simulink model "flightControlSystem"  (R2021a)
settings: Solver=ode3  StartTime=0  StopTime=TFinal  FixedStep=Ts  RelTol=1e-3  EnableMultiTasking=on
undefined symbols (not defined in the file): codertarget, Controller, DiscIntNeverNeededParam, Discrete, Estimator, g, gray, init, Sensors, Time, Ts, var_acc_angle_N, var_bias_gyr_N, var_gyro_p_N, Vehicle
libraries: simulink x39, pid_lib x4, ctrlSharedLib x4, sharedtransform x3, parrotlib x1
(part 3 of 4)

== matlab function flightControlSystem/Image Processing System/MATLAB Function ==
  data: in input; white_old input; all output; b output; x_new output; y_new output; x_old input; y_old input; change_old input; flag input; white output; flag2 input; change output; check_new output; check_old input; last input; last_old output
function [all,b,x_new,y_new,white,change,check_new,last_old] = calculate_ang(in,white_old, x_old, y_old, change_old, flag, flag2,check_old,last)
    white = 0;
    all = 0;
    red = in(:,:,1);
    filtered = imgaussfilt(red,2);
    b = imbinarize(filtered);
    for x=1:20
        for y=1:120
            b(y,x) = 0;
            b(y,(161-x)) = 0;
        end
    end
    N = 1;
    check_new = check_old;
    out = zeros(2,N);
    m00 = zeros(1,N);
    m01 = zeros(1,N);
    m10 = zeros(1,N);
    change = change_old; 
    % --------------------------------------------------------------

    if flag ~= 0
    
        m = -y_old/x_old;
        m1 = -1/m;
        %x = 1:160;
        %y = m1*x+c1;
     %----------------------------- Triangle 1
        
        x_tri1 = x_old*0.707 + y_old*-0.707;
        y_tri1 = x_old*0.707 + y_old*0.707;

        m = -y_tri1/x_tri1;
        m1 = -1/m;
        c1 = 60-80*m1;

        grad1 = m1;
        offset1 = c1;
        %[0.7071 0.7071; -0.7071 0.7071]
        x_tri2 = x_old*0.707 + y_old*0.707;
        y_tri2 = x_old*-0.707 + y_old*0.707;
        multiplier = 1;
        m = -y_tri2/x_tri2;
        m1 = -1/m;
        c1 = 60-80*m1;
        grad2 = m1;
        offset2 = c1;
        maxx = 70;
        limit = 2800;
        abs_grad = y_old/x_old;
            if abs_grad > 1 || abs_grad < -1
                if y_old > 0 
                    if x_old > 0 
                        last = 5;
                        if check_new == 0
                            change = 5;
                            if white_old ~=0
                                check_new = multiplier*maxx;
                            else
                                check_new = maxx;
                            end
                        end
                        if change ~= last
                            %change = last;
                            check_new = check_new - 1;
                        elseif change == last
                            if check_new < maxx
                                check_new = check_new + 1;
                            end
                        end
                        
                        if change == 0 %FRFC Row then Col
                            for row=1:120
                                for col=1:160
                                    if row>grad1*col + offset1 || row>grad2*col + offset2
                                        if b(row,col) == 1 && white < limit && flag2 == 1
                                            b(row,col) = 0;
                                            white = white + 1;
                                            all = all + 1;
                                        elseif b(row,col) == 1
                                            all = all + 1;
                                        end
                                    end
                                end
                            end
                        elseif change == 1  %FRFC Col then Row
                            for col=1:160
                                for row=1:120
                                    if row>grad1*col + offset1 || row>grad2*col + offset2
                                        if b(row,col) == 1 && white < limit && flag2 == 1
                                            b(row,col) = 0;
                                            white = white + 1;
                                            all = all + 1;
                                        elseif b(row,col) == 1
                                            all = all + 1;
                                        end
                                    end
                                end
                            end
                        elseif change == 2  %FRLC Row then Col
                            for row=1:120
                                for col=1:160
                                    if row>grad1*(161-col) + offset1 || row>grad2*(161-col) + offset2
                                         if b(row,(161-col)) == 1 && white < limit && flag2 == 1
                                            b(row,(161-col)) = 0;
                                            white = white + 1;
                                            all = all + 1;
                                         elseif b(row,(161-col)) == 1
                                            all = all + 1;
                                        end
                                    end
                                end
                            end
                            
                            
                         elseif change == 3  %FRLC Col then Row
                            for col=1:160
                                for row=1:120
                                    if row>grad1*(161-col) + offset1 || row>grad2*(161-col) + offset2
                                         if b(row,(161-col)) == 1 && white < limit && flag2 == 1
                                            b(row,(161-col)) = 0;
                                            white = white + 1;
                                            all = all + 1;
                                         elseif b(row,(161-col)) == 1
                                            all = all + 1;
                                        end
                                    end
                                end
                            end  
                           
                            
                          elseif change == 4  %LRFC Row then Col
                            for row=1:120
                                for col=1:160
                                    if (121-row)>grad1*col + offset1 || (121-row)>grad2*col + offset2
                                         if b((121-row),col) == 1 && white < limit && flag2 == 1
                                            b((121-row),col) = 0;
                                            white = white + 1;
                                            all = all + 1;
                                         elseif b((121-row),col) == 1
                                            all = all + 1;
                                        end
                                    end
                                end
                            end  
                            
                          elseif change == 5  %LRFC Col then Row
                            for col=1:160
                                for row=1:120
                                    if (121-row)>grad1*col + offset1 || (121-row)>grad2*col + offset2
                                         if b((121-row),col) == 1 && white < limit && flag2 == 1
                                            b((121-row),col) = 0;
                                            white = white + 1;
                                            all = all + 1;
                                         elseif b((121-row),col) == 1
                                            all = all + 1;
                                        end
                                    end
                                end
                            end  
                            
                           elseif change == 6  %LRLC Row then Col
                            for row=1:120
                                for col=1:160
                                    if (121-row)>grad1*(161-col) + offset1 || (121-row)>grad2*(161-col) + offset2
                                         if b((121-row),(161-col)) == 1 && white < limit && flag2 == 1
                                            b((121-row),(161-col)) = 0;
                                            white = white + 1;
                                            all = all + 1;
                                         elseif b((121-row),(161-col)) == 1
                                            all = all + 1;
                                        end
                                    end
                                end
                            end  
                            
                            elseif change == 7  %LRLC Col then Row
                            for col=1:160
                                for row=1:120
                                    if (121-row)>grad1*(161-col) + offset1 || (121-row)>grad2*(161-col) + offset2
                                         if b((121-row),(161-col)) == 1 && white < limit && flag2 == 1
                                            b((121-row),(161-col)) = 0;
                                            white = white + 1;
                                            all = all + 1;
                                         elseif b((121-row),(161-col)) == 1
                                            all = all + 1;
                                        end
                                    end
                                end
                            end   
                        end
                    else
                        last = 7;
                        if check_new == 0
                            if white_old ~=0
                                check_new = multiplier*maxx;
                            else
                                check_new = maxx;
                            end
                            change = 7;
                        end
                        if change ~= last
                            check_new = check_new - 1;
                            %change = last;
                        elseif change == last
                            if check_new < maxx
                                check_new = check_new + 1;
                            end
                        end
                        

                        
                        if change == 0 %FRFC Row then Col
                            for row=1:120
                                for col=1:160
                                    if row>grad1*col + offset1 || row>grad2*col + offset2
                                        if b(row,col) == 1 && white < limit && flag2 == 1
                                            b(row,col) = 0;
                                            white = white + 1;
                                            all = all + 1;
                                        elseif b(row,col) == 1
                                            all = all + 1;
                                        end
                                    end
                                end
                            end
                        elseif change == 1  %FRFC Col then Row
                            for col=1:160
                                for row=1:120
                                    if row>grad1*col + offset1 || row>grad2*col + offset2
                                        if b(row,col) == 1 && white < limit && flag2 == 1
                                            b(row,col) = 0;
                                            white = white + 1;
                                            all = all + 1;
                                        elseif b(row,col) == 1
                                            all = all + 1;
                                        end
                                    end
                                end
                            end
                        elseif change == 2  %FRLC Row then Col
                            for row=1:120
                                for col=1:160
                                    if row>grad1*(161-col) + offset1 || row>grad2*(161-col) + offset2
                                         if b(row,(161-col)) == 1 && white < limit && flag2 == 1
                                            b(row,(161-col)) = 0;
                                            white = white + 1;
                                            all = all + 1;
                                         elseif b(row,(161-col)) == 1
                                            all = all + 1;
                                        end
                                    end
                                end
                            end
                            
                            
                         elseif change == 3  %FRLC Col then Row
                            for col=1:160
                                for row=1:120
                                    if row>grad1*(161-col) + offset1 || row>grad2*(161-col) + offset2
                                         if b(row,(161-col)) == 1 && white < limit && flag2 == 1
                                            b(row,(161-col)) = 0;
                                            white = white + 1;
                                            all = all + 1;
                                         elseif b(row,(161-col)) == 1
                                            all = all + 1;
                                        end
                                    end
                                end
                            end  
                           
                            
                          elseif change == 4  %LRFC Row then Col
                            for row=1:120
                                for col=1:160
                                    if (121-row)>grad1*col + offset1 || (121-row)>grad2*col + offset2
                                         if b((121-row),col) == 1 && white < limit && flag2 == 1
                                            b((121-row),col) = 0;
                                            white = white + 1;
                                            all = all + 1;
                                         elseif b((121-row),col) == 1
                                            all = all + 1;
                                        end
                                    end
                                end
                            end  
                            
                          elseif change == 5  %LRFC Col then Row
                            for col=1:160
                                for row=1:120
                                    if (121-row)>grad1*col + offset1 || (121-row)>grad2*col + offset2
                                         if b((121-row),col) == 1 && white < limit && flag2 == 1
                                            b((121-row),col) = 0;
                                            white = white + 1;
                                            all = all + 1;
                                         elseif b((121-row),col) == 1
                                            all = all + 1;
                                        end
                                    end
                                end
                            end  
                            
                           elseif change == 6  %LRLC Row then Col
                            for row=1:120
                                for col=1:160
                                    if (121-row)>grad1*(161-col) + offset1 || (121-row)>grad2*(161-col) + offset2
                                         if b((121-row),(161-col)) == 1 && white < limit && flag2 == 1
                                            b((121-row),(161-col)) = 0;
                                            white = white + 1;
                                            all = all + 1;
                                         elseif b((121-row),(161-col)) == 1
                                            all = all + 1;
                                        end
                                    end
                                end
                            end  
                            
                            elseif change == 7  %LRLC Col then Row
                            for col=1:160
                                for row=1:120
                                    if (121-row)>grad1*(161-col) + offset1 || (121-row)>grad2*(161-col) + offset2
                                         if b((121-row),(161-col)) == 1 && white < limit && flag2 == 1
                                            b((121-row),(161-col)) = 0;
                                            white = white + 1;
                                            all = all + 1;
                                         elseif b((121-row),(161-col)) == 1
                                            all = all + 1;
                                        end
                                    end
                                end
                            end
                        end 
                    end
                else
                    if x_old > 0
                        
                        last = 1;
                        if check_new == 0
                            change = 1;
                            if white_old ~=0
                                check_new = multiplier*maxx;
                            else
                                check_new = maxx;
                            end
                        end
                        if change ~= last
                            check_new = check_new - 1;
                            %change = last;
                        elseif change == last
                            if check_new < maxx
                                check_new = check_new + 1;
                            end
                        end
                        
                        

                        if change == 0 %FRFC Row then Col
                            for row=1:120
                                for col=1:160
                                    if row<grad1*col + offset1 || row<grad2*col + offset2
                                        if b(row,col) == 1 && white < limit && flag2 == 1
                                            b(row,col) = 0;
                                            white = white + 1;
                                            all = all + 1;
                                        elseif b(row,col) == 1
                                            all = all + 1;
                                        end
                                    end
                                end
                            end
                        elseif change == 1  %FRFC Col then Row
                            for col=1:160
                                for row=1:120
                                    if row<grad1*col + offset1 || row<grad2*col + offset2
                                        if b(row,col) == 1 && white < limit && flag2 == 1
                                            b(row,col) = 0;
                                            white = white + 1;
                                            all = all + 1;
                                        elseif b(row,col) == 1
                                            all = all + 1;
                                        end
                                    end
                                end
                            end
                        elseif change == 2  %FRLC Row then Col
                            for row=1:120
                                for col=1:160
                                    if row<grad1*(161-col) + offset1 || row<grad2*(161-col) + offset2
                                         if b(row,(161-col)) == 1 && white < limit && flag2 == 1
                                            b(row,(161-col)) = 0;
                                            white = white + 1;
                                            all = all + 1;
                                         elseif b(row,(161-col)) == 1
                                            all = all + 1;
                                        end
                                    end
                                end
                            end
                            
                            
                         elseif change == 3  %FRLC Col then Row
                            for col=1:160
                                for row=1:120
                                    if row<grad1*(161-col) + offset1 || row<grad2*(161-col) + offset2
                                         if b(row,(161-col)) == 1 && white < limit && flag2 == 1
                                            b(row,(161-col)) = 0;
                                            white = white + 1;
                                            all = all + 1;
                                         elseif b(row,(161-col)) == 1
                                            all = all + 1;
                                        end
                                    end
                                end
                            end  
                           
                            
                          elseif change == 4  %LRFC Row then Col
                            for row=1:120
                                for col=1:160
                                    if (121-row)<grad1*col + offset1 || (121-row)<grad2*col + offset2
                                         if b((121-row),col) == 1 && white < limit && flag2 == 1
                                            b((121-row),col) = 0;
                                            white = white + 1;
                                            all = all + 1;
                                         elseif b((121-row),col) == 1
                                            all = all + 1;
                                        end
                                    end
                                end
                            end  
                            
                          elseif change == 5  %LRFC Col then Row
                            for col=1:160
                                for row=1:120
                                    if (121-row)<grad1*col + offset1 || (121-row)<grad2*col + offset2
                                         if b((121-row),col) == 1 && white < limit && flag2 == 1
                                            b((121-row),col) = 0;
                                            white = white + 1;
                                            all = all + 1;
                                         elseif b((121-row),col) == 1
                                            all = all + 1;
                                        end
                                    end
                                end
                            end  
                            
                           elseif change == 6  %LRLC Row then Col
                            for row=1:120
                                for col=1:160
                                    if (121-row)<grad1*(161-col) + offset1 || (121-row)<grad2*(161-col) + offset2
                                         if b((121-row),(161-col)) == 1 && white < limit && flag2 == 1
                                            b((121-row),(161-col)) = 0;
                                            white = white + 1;
                                            all = all + 1;
                                         elseif b((121-row),(161-col)) == 1
                                            all = all + 1;
                                        end
                                    end
                                end
                            end  
                            
                            elseif change == 7  %LRLC Col then Row
                            for col=1:160
                                for row=1:120
                                    if (121-row)<grad1*(161-col) + offset1 || (121-row)<grad2*(161-col) + offset2
                                         if b((121-row),(161-col)) == 1 && white < limit && flag2 == 1
                                            b((121-row),(161-col)) = 0;
                                            white = white + 1;
                                            all = all + 1;
                                         elseif b((121-row),(161-col)) == 1
                                            all = all + 1;
                                        end
                                    end
                                end
                            end
                        end  
                        
                        
 
                        
                        
                    else
                        
                        last = 3;
                        if check_new == 0
                            change = 3;
                            if white_old ~=0
                                check_new = multiplier*maxx;
                            else
                                check_new = maxx;
                            end
                        end
                        if change ~= last
                            check_new = check_new - 1;
                            %change = last;
                        elseif change == last
                            if check_new < maxx
                                check_new = check_new + 1;
                            end
                        end
                        
                        
                        
                        
                        if change == 0 %FRFC Row then Col
                            for row=1:120
                                for col=1:160
                                    if row<grad1*col + offset1 || row<grad2*col + offset2
                                        if b(row,col) == 1 && white < limit && flag2 == 1
                                            b(row,col) = 0;
                                            white = white + 1;
                                            all = all + 1;
                                        elseif b(row,col) == 1
                                            all = all + 1;
                                        end
                                    end
                                end
                            end
                        elseif change == 1  %FRFC Col then Row
                            for col=1:160
                                for row=1:120
                                    if row<grad1*col + offset1 || row<grad2*col + offset2
                                        if b(row,col) == 1 && white < limit && flag2 == 1
                                            b(row,col) = 0;
                                            white = white + 1;
                                            all = all + 1;
                                        elseif b(row,col) == 1
                                            all = all + 1;
                                        end
                                    end
                                end
                            end
                        elseif change == 2  %FRLC Row then Col
                            for row=1:120
                                for col=1:160
                                    if row<grad1*(161-col) + offset1 || row<grad2*(161-col) + offset2
                                         if b(row,(161-col)) == 1 && white < limit && flag2 == 1
                                            b(row,(161-col)) = 0;
                                            white = white + 1;
                                            all = all + 1;
                                         elseif b(row,(161-col)) == 1
                                            all = all + 1;
                                        end
                                    end
                                end
                            end
                            
                            
                         elseif change == 3  %FRLC Col then Row
                            for col=1:160
                                for row=1:120
                                    if row<grad1*(161-col) + offset1 || row<grad2*(161-col) + offset2
                                         if b(row,(161-col)) == 1 && white < limit && flag2 == 1
                                            b(row,(161-col)) = 0;
                                            white = white + 1;
                                            all = all + 1;
                                         elseif b(row,(161-col)) == 1
                                            all = all + 1;
                                        end
                                    end
                                end
                            end  
                           
                            
                          elseif change == 4  %LRFC Row then Col
                            for row=1:120
                                for col=1:160
                                    if (121-row)<grad1*col + offset1 || (121-row)<grad2*col + offset2
                                         if b((121-row),col) == 1 && white < limit && flag2 == 1
                                            b((121-row),col) = 0;
                                            white = white + 1;
                                            all = all + 1;
                                         elseif b((121-row),col) == 1
                                            all = all + 1;
                                        end
                                    end
                                end
                            end  
                            
                          elseif change == 5  %LRFC Col then Row
                            for col=1:160
                                for row=1:120
                                    if (121-row)<grad1*col + offset1 || (121-row)<grad2*col + offset2
                                         if b((121-row),col) == 1 && white < limit && flag2 == 1
                                            b((121-row),col) = 0;
                                            white = white + 1;
                                            all = all + 1;
                                         elseif b((121-row),col) == 1
                                            all = all + 1;
                                        end
                                    end
                                end
                            end  
                            
                           elseif change == 6  %LRLC Row then Col
                            for row=1:120
                                for col=1:160
                                    if (121-row)<grad1*(161-col) + offset1 || (121-row)<grad2*(161-col) + offset2
                                         if b((121-row),(161-col)) == 1 && white < limit && flag2 == 1
                                            b((121-row),(161-col)) = 0;
                                            white = white + 1;
                                            all = all + 1;
                                         elseif b((121-row),(161-col)) == 1
                                            all = all + 1;
                                        end
                                    end
                                end
                            end  
                            
                            elseif change == 7  %LRLC Col then Row
                            for col=1:160
                                for row=1:120
                                    if (121-row)<grad1*(161-col) + offset1 || (121-row)<grad2*(161-col) + offset2
                                         if b((121-row),(161-col)) == 1 && white < limit && flag2 == 1
                                            b((121-row),(161-col)) = 0;
                                            white = white + 1;
                                            all = all + 1;
                                         elseif b((121-row),(161-col)) == 1
                                            all = all + 1;
                                        end
                                    end
                                end
                            end
                        end 
                                     
                        
                    end
                end
            else
                if x_old > 0
                    if y_old < 0
                        last = 0;
                        if check_new == 0
                            change = 0;
                            if white_old ~=0
                                check_new = multiplier*maxx;
                            else
                                check_new = maxx;
                            end
                        end
                        if change ~= last
                            %change = last;
                            check_new = check_new - 1;
                        elseif change == last
                            if check_new < maxx
                                check_new = check_new + 1;
                            end
                        end
                        
                        
                        
                        
                        if change == 0 %FRFC Row then Col
                            for row=1:120
                                for col=1:160
                                    if row>grad1*col + offset1 || row<grad2*col + offset2
                                        if b(row,col) == 1 && white < limit && flag2 == 1
                                            b(row,col) = 0;
                                            white = white + 1;
                                            all = all + 1;
                                        elseif b(row,col) == 1
                                            all = all + 1;
                                        end
                                    end
                                end
                            end
                        elseif change == 1  %FRFC Col then Row
                            for col=1:160
                                for row=1:120
                                    if row>grad1*col + offset1 || row<grad2*col + offset2
                                        if b(row,col) == 1 && white < limit && flag2 == 1
                                            b(row,col) = 0;
                                            white = white + 1;
                                            all = all + 1;
                                        elseif b(row,col) == 1
                                            all = all + 1;
                                        end
                                    end
                                end
                            end
                        elseif change == 2  %FRLC Row then Col
                            for row=1:120
                                for col=1:160
                                    if row>grad1*(161-col) + offset1 || row<grad2*(161-col) + offset2
                                         if b(row,(161-col)) == 1 && white < limit && flag2 == 1
                                            b(row,(161-col)) = 0;
                                            white = white + 1;
                                            all = all + 1;
                                         elseif b(row,(161-col)) == 1
                                            all = all + 1;
                                        end
                                    end
                                end
                            end
                            
                            
                         elseif change == 3  %FRLC Col then Row
                            for col=1:160
                                for row=1:120
                                    if row>grad1*(161-col) + offset1 || row<grad2*(161-col) + offset2
                                         if b(row,(161-col)) == 1 && white < limit && flag2 == 1
                                            b(row,(161-col)) = 0;
                                            white = white + 1;
                                            all = all + 1;
                                         elseif b(row,(161-col)) == 1
                                            all = all + 1;
                                        end
                                    end
                                end
                            end  
                           
                            
                          elseif change == 4  %LRFC Row then Col
                            for row=1:120
                                for col=1:160
                                    if (121-row)>grad1*col + offset1 || (121-row)<grad2*col + offset2
                                         if b((121-row),col) == 1 && white < limit && flag2 == 1
                                            b((121-row),col) = 0;
                                            white = white + 1;
                                            all = all + 1;
                                         elseif b((121-row),col) == 1
                                            all = all + 1;
                                        end
                                    end
                                end
                            end  
                            
                          elseif change == 5  %LRFC Col then Row
                            for col=1:160
                                for row=1:120
                                    if (121-row)>grad1*col + offset1 || (121-row)<grad2*col + offset2
                                         if b((121-row),col) == 1 && white < limit && flag2 == 1
                                            b((121-row),col) = 0;
                                            white = white + 1;
                                            all = all + 1;
                                         elseif b((121-row),col) == 1
                                            all = all + 1;
                                        end
                                    end
                                end
                            end  
                            
                           elseif change == 6  %LRLC Row then Col
                            for row=1:120
                                for col=1:160
                                    if (121-row)>grad1*(161-col) + offset1 || (121-row)<grad2*(161-col) + offset2
                                         if b((121-row),(161-col)) == 1 && white < limit && flag2 == 1
                                            b((121-row),(161-col)) = 0;
                                            white = white + 1;
                                            all = all + 1;
                                         elseif b((121-row),(161-col)) == 1
                                            all = all + 1;
                                        end
                                    end
                                end
                            end  
                            
                            elseif change == 7  %LRLC Col then Row
                            for col=1:160
                                for row=1:120
                                    if (121-row)>grad1*(161-col) + offset1 || (121-row)<grad2*(161-col) + offset2
                                         if b((121-row),(161-col)) == 1 && white < limit && flag2 == 1
                                            b((121-row),(161-col)) = 0;
                                            white = white + 1;
                                            all = all + 1;
                                         elseif b((121-row),(161-col)) == 1
                                            all = all + 1;
                                        end
                                    end
                                end
                            end
                        end 
                        
                        
                        
                        
                        
                    else
                        
                        last = 4;
                        if check_new == 0
                            change = 4;
                            if white_old ~=0
                                check_new = multiplier*maxx;
                            else
                                check_new = maxx;
                            end
                        end
                        if change ~= last
                            %change = last;
                            check_new = check_new - 1;
                        elseif change == last
                            if check_new < maxx
                                check_new = check_new + 1;
                            end
                        end
                        
                        if change == 0 %FRFC Row then Col
                            for row=1:120
                                for col=1:160
                                    if row>grad1*col + offset1 || row<grad2*col + offset2
                                        if b(row,col) == 1 && white < limit && flag2 == 1
                                            b(row,col) = 0;
                                            white = white + 1;
                                            all = all + 1;
                                        elseif b(row,col) == 1
                                            all = all + 1;
                                        end
                                    end
                                end
                            end
                        elseif change == 1  %FRFC Col then Row
                            for col=1:160
                                for row=1:120
                                    if row>grad1*col + offset1 || row<grad2*col + offset2
                                        if b(row,col) == 1 && white < limit && flag2 == 1
                                            b(row,col) = 0;
                                            white = white + 1;
                                            all = all + 1;
                                        elseif b(row,col) == 1
                                            all = all + 1;
                                        end
                                    end
                                end
                            end
                        elseif change == 2  %FRLC Row then Col
                            for row=1:120
                                for col=1:160
                                    if row>grad1*(161-col) + offset1 || row<grad2*(161-col) + offset2
                                         if b(row,(161-col)) == 1 && white < limit && flag2 == 1
                                            b(row,(161-col)) = 0;
                                            white = white + 1;
                                            all = all + 1;
                                         elseif b(row,(161-col)) == 1
                                            all = all + 1;
                                        end
                                    end
                                end
                            end
                            
                            
                         elseif change == 3  %FRLC Col then Row
                            for col=1:160
                                for row=1:120
                                    if row>grad1*(161-col) + offset1 || row<grad2*(161-col) + offset2
                                         if b(row,(161-col)) == 1 && white < limit && flag2 == 1
                                            b(row,(161-col)) = 0;
                                            white = white + 1;
                                            all = all + 1;
                                         elseif b(row,(161-col)) == 1
                                            all = all + 1;
                                        end
                                    end
                                end
                            end  
                           
                            
                          elseif change == 4  %LRFC Row then Col
                            for row=1:120
                                for col=1:160
                                    if (121-row)>grad1*col + offset1 || (121-row)<grad2*col + offset2
                                         if b((121-row),col) == 1 && white < limit && flag2 == 1
                                            b((121-row),col) = 0;
                                            white = white + 1;
                                            all = all + 1;
                                         elseif b((121-row),col) == 1
                                            all = all + 1;
                                        end
                                    end
                                end
                            end  
                            
                          elseif change == 5  %LRFC Col then Row
                            for col=1:160
                                for row=1:120
                                    if (121-row)>grad1*col + offset1 || (121-row)<grad2*col + offset2
                                         if b((121-row),col) == 1 && white < limit && flag2 == 1
                                            b((121-row),col) = 0;
                                            white = white + 1;
                                            all = all + 1;
                                         elseif b((121-row),col) == 1
                                            all = all + 1;
                                        end
                                    end
                                end
                            end  
                            
                           elseif change == 6  %LRLC Row then Col
                            for row=1:120
                                for col=1:160
                                    if (121-row)>grad1*(161-col) + offset1 || (121-row)<grad2*(161-col) + offset2
                                         if b((121-row),(161-col)) == 1 && white < limit && flag2 == 1
                                            b((121-row),(161-col)) = 0;
                                            white = white + 1;
                                            all = all + 1;
                                         elseif b((121-row),(161-col)) == 1
                                            all = all + 1;
                                        end
                                    end
                                end
                            end  
                            
                            elseif change == 7  %LRLC Col then Row
                            for col=1:160
                                for row=1:120
                                    if (121-row)>grad1*(161-col) + offset1 || (121-row)<grad2*(161-col) + offset2
                                         if b((121-row),(161-col)) == 1 && white < limit && flag2 == 1
                                            b((121-row),(161-col)) = 0;
                                            white = white + 1;
                                            all = all + 1;
                                         elseif b((121-row),(161-col)) == 1
                                            all = all + 1;
                                        end
                                    end
                                end
                            end
                        end           
                   
                    end
                else
                    if y_old < 0
                        
                        last = 2;
                        if check_new == 0
                            change = 2;
                            if white_old ~=0
                                check_new = multiplier*maxx;
                            else
                                check_new = maxx;
                            end
                        end
                        if change ~= last
                            %change = last;
                            check_new = check_new - 1;
                        elseif change == last
                            if check_new < maxx
                                check_new = check_new + 1;
                            end
                        end
                        
                        if change == 0 %FRFC Row then Col
                            for row=1:120
                                for col=1:160
                                    if row<grad1*col + offset1 || row>grad2*col + offset2
                                        if b(row,col) == 1 && white < limit && flag2 == 1
                                            b(row,col) = 0;
                                            white = white + 1;
                                            all = all + 1;
                                        elseif b(row,col) == 1
                                            all = all + 1;
                                        end
                                    end
                                end
                            end
                        elseif change == 1  %FRFC Col then Row
                            for col=1:160
                                for row=1:120
                                    if row<grad1*col + offset1 || row>grad2*col + offset2
                                        if b(row,col) == 1 && white < limit && flag2 == 1
                                            b(row,col) = 0;
                                            white = white + 1;
                                            all = all + 1;
                                        elseif b(row,col) == 1
                                            all = all + 1;
                                        end
                                    end
                                end
                            end
                        elseif change == 2  %FRLC Row then Col
                            for row=1:120
                                for col=1:160
                                    if row<grad1*(161-col) + offset1 || row>grad2*(161-col) + offset2
                                         if b(row,(161-col)) == 1 && white < limit && flag2 == 1
                                            b(row,(161-col)) = 0;
                                            white = white + 1;
                                            all = all + 1;
                                         elseif b(row,(161-col)) == 1
                                            all = all + 1;
                                        end
                                    end
                                end
                            end
                            
                            
                         elseif change == 3  %FRLC Col then Row
                            for col=1:160
                                for row=1:120
                                    if row<grad1*(161-col) + offset1 || row>grad2*(161-col) + offset2
                                         if b(row,(161-col)) == 1 && white < limit && flag2 == 1
                                            b(row,(161-col)) = 0;
                                            white = white + 1;
                                            all = all + 1;
                                         elseif b(row,(161-col)) == 1
                                            all = all + 1;
                                        end
                                    end
                                end
                            end  
                           
                            
                          elseif change == 4  %LRFC Row then Col
                            for row=1:120
                                for col=1:160
                                    if (121-row)<grad1*col + offset1 || (121-row)>grad2*col + offset2
                                         if b((121-row),col) == 1 && white < limit && flag2 == 1
                                            b((121-row),col) = 0;
                                            white = white + 1;
                                            all = all + 1;
                                         elseif b((121-row),col) == 1
                                            all = all + 1;
                                        end
                                    end
                                end
                            end  
                            
                          elseif change == 5  %LRFC Col then Row
                            for col=1:160
                                for row=1:120
                                    if (121-row)<grad1*col + offset1 || (121-row)>grad2*col + offset2
                                         if b((121-row),col) == 1 && white < limit && flag2 == 1
                                            b((121-row),col) = 0;
                                            white = white + 1;
                                            all = all + 1;
                                         elseif b((121-row),col) == 1
                                            all = all + 1;
                                        end
                                    end
                                end
                            end  
                            
                           elseif change == 6  %LRLC Row then Col
                            for row=1:120
                                for col=1:160
                                    if (121-row)<grad1*(161-col) + offset1 || (121-row)>grad2*(161-col) + offset2
                                         if b((121-row),(161-col)) == 1 && white < limit && flag2 == 1
                                            b((121-row),(161-col)) = 0;
                                            white = white + 1;
                                            all = all + 1;
                                         elseif b((121-row),(161-col)) == 1
                                            all = all + 1;
                                        end
                                    end
                                end
                            end  
                            
                            elseif change == 7  %LRLC Col then Row
                            for col=1:160
                                for row=1:120
                                    if (121-row)<grad1*(161-col) + offset1 || (121-row)>grad2*(161-col) + offset2
                                         if b((121-row),(161-col)) == 1 && white < limit && flag2 == 1
                                            b((121-row),(161-col)) = 0;
                                            white = white + 1;
                                            all = all + 1;
                                         elseif b((121-row),(161-col)) == 1
                                            all = all + 1;
                                        end
                                    end
                                end
                            end
                        end 
                       
                        
                    else
                        last = 6;
                        if check_new == 0
                            change = 6;
                            if white_old ~=0
                                check_new = multiplier*maxx;
                            else
                                check_new = maxx;
                            end
                        end
                        if change ~= last
                            check_new = check_new - 1;
                            %change = last;
                        elseif change == last
                            if check_new < maxx
                                check_new = check_new + 1;
                            end
                        end
                        
                        if change == 0 %FRFC Row then Col
                            for row=1:120
                                for col=1:160
                                    if row<grad1*col + offset1 || row>grad2*col + offset2
                                        if b(row,col) == 1 && white < limit && flag2 == 1
                                            b(row,col) = 0;
                                            white = white + 1;
                                            all = all + 1;
                                        elseif b(row,col) == 1
                                            all = all + 1;
                                        end
                                    end
                                end
                            end
                        elseif change == 1  %FRFC Col then Row
                            for col=1:160
                                for row=1:120
                                    if row<grad1*col + offset1 || row>grad2*col + offset2
                                        if b(row,col) == 1 && white < limit && flag2 == 1
                                            b(row,col) = 0;
                                            white = white + 1;
                                            all = all + 1;
                                        elseif b(row,col) == 1
                                            all = all + 1;
                                        end
                                    end
                                end
                            end
                        elseif change == 2  %FRLC Row then Col
                            for row=1:120
                                for col=1:160
                                    if row<grad1*(161-col) + offset1 || row>grad2*(161-col) + offset2
                                         if b(row,(161-col)) == 1 && white < limit && flag2 == 1
                                            b(row,(161-col)) = 0;
                                            white = white + 1;
                                            all = all + 1;
                                         elseif b(row,(161-col)) == 1
                                            all = all + 1;
                                        end
                                    end
                                end
                            end
                            
                            
                         elseif change == 3  %FRLC Col then Row
                            for col=1:160
                                for row=1:120
                                    if row<grad1*(161-col) + offset1 || row>grad2*(161-col) + offset2
                                         if b(row,(161-col)) == 1 && white < limit && flag2 == 1
                                            b(row,(161-col)) = 0;
                                            white = white + 1;
                                            all = all + 1;
                                         elseif b(row,(161-col)) == 1
                                            all = all + 1;
                                        end
                                    end
                                end
                            end  
                           
                            
                          elseif change == 4  %LRFC Row then Col
                            for row=1:120
                                for col=1:160
                                    if (121-row)<grad1*col + offset1 || (121-row)>grad2*col + offset2
                                         if b((121-row),col) == 1 && white < limit && flag2 == 1
                                            b((121-row),col) = 0;
                                            white = white + 1;
                                            all = all + 1;
                                         elseif b((121-row),col) == 1
                                            all = all + 1;
                                        end
                                    end
                                end
                            end  
                            
                          elseif change == 5  %LRFC Col then Row
                            for col=1:160
                                for row=1:120
                                    if (121-row)<grad1*col + offset1 || (121-row)>grad2*col + offset2
                                         if b((121-row),col) == 1 && white < limit && flag2 == 1
                                            b((121-row),col) = 0;
                                            white = white + 1;
                                            all = all + 1;
                                         elseif b((121-row),col) == 1
                                            all = all + 1;
                                        end
                                    end
                                end
                            end  
                            
                           elseif change == 6  %LRLC Row then Col
                            for row=1:120
                                for col=1:160
                                    if (121-row)<grad1*(161-col) + offset1 || (121-row)>grad2*(161-col) + offset2
                                         if b((121-row),(161-col)) == 1 && white < limit && flag2 == 1
                                            b((121-row),(161-col)) = 0;
                                            white = white + 1;
                                            all = all + 1;
                                         elseif b((121-row),(161-col)) == 1
                                            all = all + 1;
                                        end
                                    end
                                end
                            end  
                            
                            elseif change == 7  %LRLC Col then Row
                            for col=1:160
                                for row=1:120
                                    if (121-row)<grad1*(161-col) + offset1 || (121-row)>grad2*(161-col) + offset2
                                         if b((121-row),(161-col)) == 1 && white < limit && flag2 == 1
                                            b((121-row),(161-col)) = 0;
                                            white = white + 1;
                                            all = all + 1;
                                         elseif b((121-row),(161-col)) == 1
                                            all = all + 1;
                                        end
                                    end
                                end
                            end
                        end
                 
                    end
                end
            end    
    end
    
    input = b;
   
    % --------------------------------------------------------------
 
    

    for row=1:120
        for col=1:160
           if input(row,col) ~=0 % on object pixel
               m10(input(row,col)) = row*1+m10(input(row,col)); 
               m01(input(row,col)) = col*1+m01(input(row,col));
               m00(input(row,col)) = m00(input(row,col)) + 1;
           end
        end
    end
    for i = 1:N
        out(2,i) = m10(i)/m00(i);
        out(1,i) = m01(i)/m00(i);
    end
    
    
    last_old = last;
    x_new = out(1,1);
    y_new = out(2,1);
    x_new = x_new - 80;
    y_new = 60-y_new;
end
